simulink model "Beta_Estimation_OpenLoop"  (R2022b)
settings: Solver=FixedStepAuto  StartTime=0.0  StopTime=t_l*0.8  FixedStep=Ts  RelTol=1e-3
settings Model: Creator=LDW  LastModifiedBy=LDW

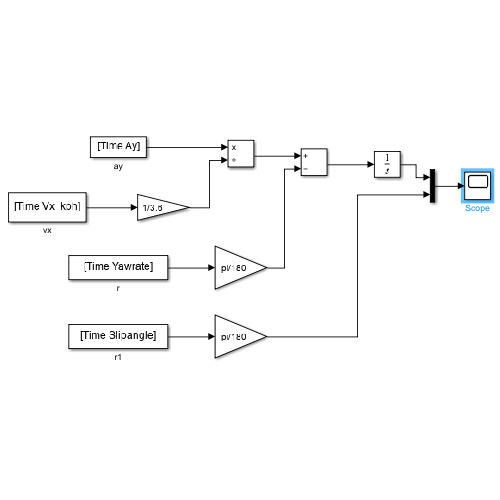
[thumbnail: Simulink's stored preview of the top-level diagram]
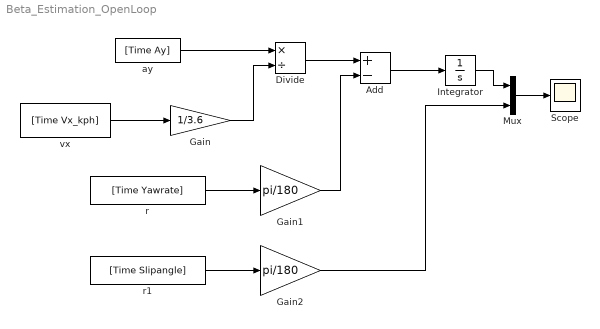
== system Beta_Estimation_OpenLoop ==
  Add : Sum  Inputs=+-
  Divide : Product  Inputs=*/
  Gain : Gain  Gain=1/3.6
  Gain1 : Gain  Gain=pi/180
  Gain2 : Gain  Gain=pi/180
  Integrator : Integrator
  Mux : Mux  Inputs=2
  Scope : Scope
  ay : FromWorkspace  VariableName=[Time Ay]
  r : FromWorkspace  VariableName=[Time Yawrate]
  r1 : FromWorkspace  VariableName=[Time Slipangle]
  vx : FromWorkspace  VariableName=[Time Vx_kph]
  wires:
  ay/1 -> Divide/1
  Divide/1 -> Add/1
  Add/1 -> Integrator/1
  Integrator/1 -> Mux/1
  Mux/1 -> Scope/1
  vx/1 -> Gain/1
  Gain/1 -> Divide/2
  r/1 -> Gain1/1
  Gain1/1 -> Add/2
  r1/1 -> Gain2/1
  Gain2/1 -> Mux/2
